simulink model "sldemo_mrv_sig_filter1_prototype"  (Simulink 7.6)
settings: Solver=FixedStepDiscrete  StartTime=0.0  StopTime=10.0  RelTol=1e-3
settings Model: Creator=The MathWorks Inc.
settings OptimizationCC: InlineParams=on
settings ModelReferenceCC: ModelReferenceNumInstancesAllowed=Single
settings RTWCC: ProcessScript=grt_make_rtw_hook
settings CodeAppCC: MaxIdLength=100

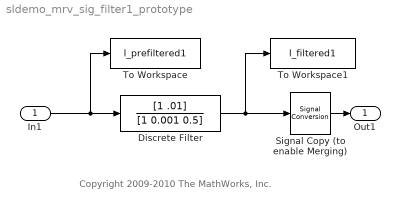
== system sldemo_mrv_sig_filter1_prototype ==
  note: Copyright 2009-2010 The MathWorks, Inc.
  In1 : Inport
  Discrete Filter : DiscreteFilter  Numerator=[1 .01]  Denominator=[1 0.001 0.5]  SampleTime=.01
  Signal Copy (to enable Merging) : SignalConversion  ConversionOutput=Contiguous copy
  To Workspace : ToWorkspace  VariableName=l_prefiltered1  SampleTime=-1  SaveFormat=Structure
  To Workspace1 : ToWorkspace  VariableName=l_filtered1  SampleTime=-1  SaveFormat=Structure
  Out1 : Outport
  wires:
  In1/1 -> Discrete Filter/1, To Workspace/1
  Discrete Filter/1 -> To Workspace1/1, Signal Copy (to enable Merging)/1
  Signal Copy (to enable Merging)/1 -> Out1/1
